simulink model "stateflow_junction"  (R2015b)
settings: Solver=VariableStepAuto  StartTime=0.0  StopTime=10.0  RelTol=1e-3
settings Model: Creator=ladmin  LastModifiedBy=ladmin

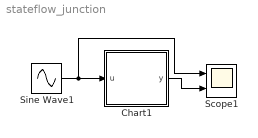
== system stateflow_junction ==
  Chart1 : Stateflow chart  TreatAsAtomicUnit=on
  Scope1 : Scope  NumInputPorts=2
  Sine Wave1 : Sin  SampleTime=0
  wires:
  Chart1/1(y) -> Scope1/2
  Sine Wave1/1 -> Scope1/1, Chart1/1(u)

== stateflow chart stateflow_junction/Chart1 ==
  state ON
    entry: y=1;
  state OFF
    entry: y=-1;
  state VERY_OFF [group]
    entry: y=-3;
  state UNKNOWN
    entry: y=0
  note: history junction
  (junction 24) -> VERY_OFF : [u<-3]
  (default) -> ON [order 1]
  (junction 15) -> (junction 24) [order 2]
  (junction 15) -> OFF [order 1] : [0<u<-3]
  ON -> (junction 15) [order 1]
  OFF -> ON [order 2] : [u>0]
  ON -> UNKNOWN [order 2] : {u=0}
  OFF -> (history) [order 1] : [u=0]
  VERY_OFF -> (history) : {u=0}
  (default) -> UNKNOWN [order 2]
  data: u input; y output
